simulink model "DoublePendulumPM"  (R2023b)
settings: Solver=FixedStepAuto  StartTime=0.0  StopTime=5  FixedStep=0.0001  RelTol=1e-3
values from neighbouring files (symbols this model uses):
  an1 = pm.Constants.r_0 / pm.Constants.l_1    [Constants.m]    (also in DoublePendulumPM_ParamSet.m = 1.5)
  an2 = pm.Constants.r_0 / pm.Constants.l_2    [Constants.m]    (also in DoublePendulumPM_ParamSet.m = 3)
  cn1 = pm.Constants.c_1 / (pm.Constants.m_1 * pm.Constants.l_1^2)    [Constants.m]    (also in DoublePendulumPM_ParamSet.m = 0.025)
  cn2 = pm.Constants.c_2 / (pm.Constants.m_2 * pm.Constants.l_2^2)    [Constants.m]    (also in DoublePendulumPM_ParamSet.m = 0.1)
  dt = 0.01    [Constants.m]    (also in DoublePendulumPM_ParamSet.m)
  l_1 = 0.2    [Constants.m]    (also in DoublePendulumPM_ParamSet.m)
  l_2 = 0.1    [Constants.m]    (also in DoublePendulumPM_ParamSet.m)
  m_1 = 1    [Constants.m]    (also in DoublePendulumPM_ParamSet.m)
  m_2 = 1    [Constants.m]    (also in DoublePendulumPM_ParamSet.m)
  N = 181    [Constants.m]
  r_0 = 0.3    [Constants.m]    (also in DoublePendulumPM_ParamSet.m)
  s = [10000.0; 10000.0; 80000.0; 5000.0; 80000.0; 5000.0]    [Constants.m]
  wn1 = pm.Constants.g   / pm.Constants.l_1    [Constants.m]    (also in DoublePendulumPM_ParamSet.m = 49.03325)
  wn2 = pm.Constants.g   / pm.Constants.l_2    [Constants.m]    (also in DoublePendulumPM_ParamSet.m = 98.0665)
undefined symbols (not defined in the file or in its folder): L, X, Y, Z
libraries: sm_lib x28, nesl_utility x9
settings Model: Creator=s0612  LastModifiedBy=0484476

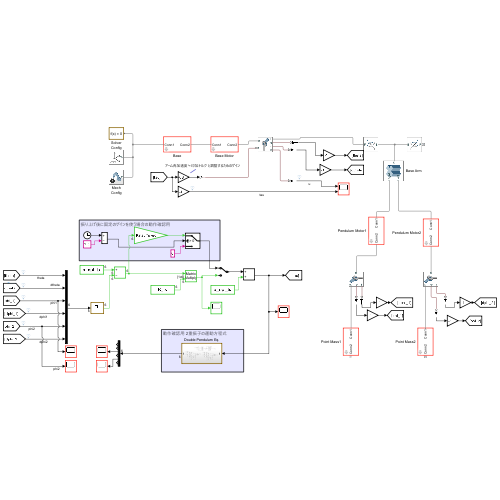
[thumbnail: Simulink's stored preview of the top-level diagram]
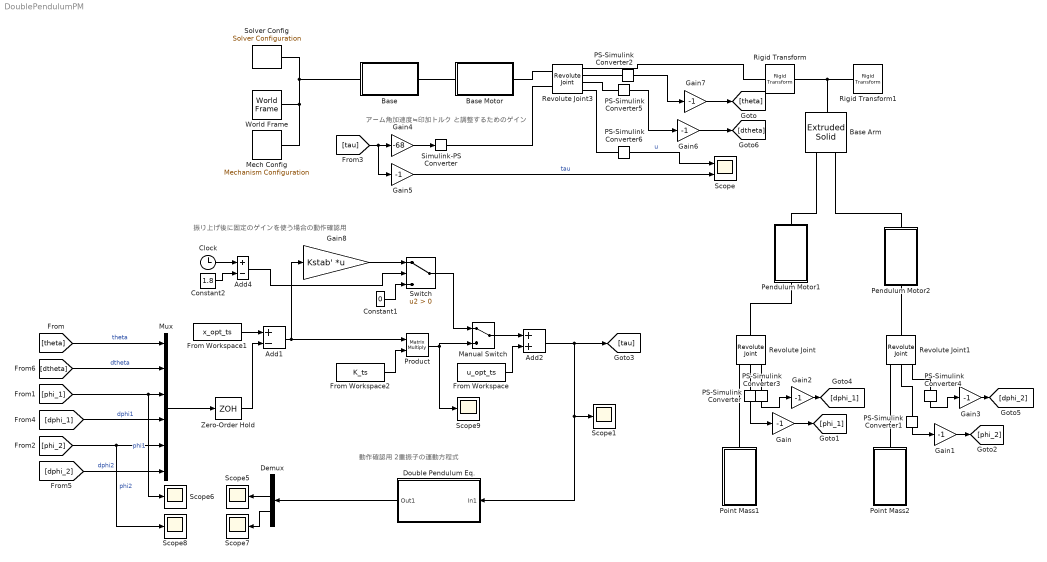
== system DoublePendulumPM ==
  note: アーム角加速度≒印加トルク と調整するためのゲイン
  note: 動作確認用 2重振子の運動方程式
  note: 振り上げ後に固定のゲインを使う場合の動作確認用
  Add1 : Sum  Inputs=+-
  Add2 : Sum
  Add4 : Sum  Inputs=+-
  Base : Subsystem  mask{L=0.2, R=0.2, rho=1000, rgb=[0.5 0.5 0.5]}
      mask prompts: L "Length[m]"; R "Radius[m]"; rho "Density[kg/m^3]"; rgb "Color (R G B)"
      mask DialogControl ParameterGroupVar Prompt: パラメーター
  Base Arm : sm_lib/Body Elements/Extruded Solid  GraphicAmbientColor=[0.15 0.15 0.15 1.0]  BasedOnType=Density  CenterOfMass=[0 0 0]  CenterOfMassUnits=m  GraphicDiffuseColor=[0.5 0.5 0.5]  ExportConvexHullGeometry=off  ExtrusionCrossSection=[r_0 0.04; 0 0.06; -r_0 0.04; -r_0 -0.04; 0 -0.06; r_0 -0.04]  ExtrusionCrossSectionUnits=m  Density=1000*1000  DensityUnits=kg/m^3  DoExposeReferenceFrame=on  GraphicEmissiveColor=[0.0 0.0 0.0 1.0]  ExportEntireGeometry=off  ExtrusionLength=0.04  ExtrusionLengthUnits=m  ExtrusionType=General  SerializedFrames=<Frames><Frame><Id>Frame1</Id><Value><Name>Right</Name><Origin><Source>GeometricFeature</Source><FeatureName>side surface 6</FeatureName></Origin><PrimaryAxis><DefinedDirection>+Z</DefinedDirection><Source>ReferenceFrame</Source><SourceDirection>+X</SourceDirection><FeatureName></FeatureName></PrimaryAxis><SecondaryAxis><DefinedDirection>+Y</DefinedDirection><Source>ReferenceFrame</Source><SourceDirection>+Y</SourceDirection><FeatureName></FeatureName></SecondaryAxis></Value></Frame><Frame><Id>Frame2</Id><Value><Name>Left</Name><Origin><Source>GeometricFeature</Source><FeatureName>side surface 3</FeatureName></Origin><PrimaryAxis><DefinedDirection>+Z</DefinedDirection><Source>ReferenceFrame</Source><SourceDirection>-X</SourceDirection><FeatureName></FeatureName></PrimaryAxis><SecondaryAxis><DefinedDirection>+Y</DefinedDirection><Source>ReferenceFrame</Source><SourceDirection>-Y</SourceDirection><FeatureName></FeatureName></SecondaryAxis></Value></Frame></Frames>  MarkerShape=Sphere  MarkerSize=10  GraphicType=FromGeometry  InertiaType=CalculateFromGeometry  Mass=1  MassUnits=kg  MomentsOfInertia=[1 1 1]  MomentsOfInertiaUnits=kg*m^2  PolygonNumSides=6  GraphicOpacity=1.0  PolygonOuterRadius=1  PolygonOuterRadiusUnits=m  ProductsOfInertia=[0 0 0]  ProductsOfInertiaUnits=kg*m^2  GraphicShininess=75  GraphicSpecularColor=[0.5 0.5 0.5 1.0]  GraphicVisPropType=SimpleVisualProperties
  Base Motor : Subsystem  mask{L=0.02, R=0.1, rho=1000, rgb=[0.5 0.5 0]}
      mask prompts: L "Length[m]"; R "Radius[m]"; rho "Density[kg/m^3]"; rgb "Color (R G B)"
      mask DialogControl ParameterGroupVar Prompt: パラメーター
  Clock : Clock
  Constant1 : Constant  Value=0
  Constant2 : Constant  Value=1.8
  Demux : Demux  Outputs=6
  Double Pendulum Eq. : Subsystem
  From Workspace : FromWorkspace  VariableName=u_opt_ts  SampleTime=0.01
  From Workspace1 : FromWorkspace  VariableName=x_opt_ts  SampleTime=dt  OutputAfterFinalValue=Holding final value
  From Workspace2 : FromWorkspace  VariableName=K_ts  SampleTime=dt  OutputAfterFinalValue=Holding final value
  Gain{,1..3,5..7} (7 alike) : Gain  Gain=-1
  Gain4 : Gain  Gain=-68
  Gain8 : Gain  Gain=Kstab'  Multiplication=Matrix(K*u) (u vector)
  Manual Switch : ManualSwitch
  Mech Config : sm_lib/Utilities/Mechanism Configuration  UniformGravity=Constant  GravityVector=[0 0 -9.80665]  GravityVectorUnits=m/s^2  LinearizationDelta=0.001  JointModeTransitionNonlinearIterations=2
  Mux : Mux  Inputs=6
  PS-Simulink Converter{,1..6} (7 alike) : nesl_utility/PS-Simulink Converter  PhysicalDomain=network_engine_domain  SubClassName=ps_output  LeftPortType=input  RightPortType=output  PseudoPeriodic=off  Frequencies=[]  VectorFormat=inherit  Unit=inherit  AffineConversion=off
  Pendulum Motor1 : Subsystem  mask{L=0.005, R=0.02, rho=0, rgb=[0.5 0.5 0]}
      mask prompts: L "Length[m]"; R "Radius[m]"; rho "Density[kg/m^3]"; rgb "Color (R G B)"
      mask DialogControl ParameterGroupVar Prompt: パラメーター
  Pendulum Motor2 : Subsystem  mask{L=0.005, R=0.02, rho=0, rgb=[0.5 0.5 0]}
      mask prompts: L "Length[m]"; R "Radius[m]"; rho "Density[kg/m^3]"; rgb "Color (R G B)"
      mask DialogControl ParameterGroupVar Prompt: パラメーター
  Point Mass1 : Subsystem  mask{L=l_1, M=m_1, rgb=[1 0.5 0]}
      mask prompts: L "Length[m]"; M "Weight[kg]"; rgb "Color (R G B)"
      mask DialogControl ParameterGroupVar Prompt: パラメーター
  Point Mass2 : Subsystem  mask{L=l_2, M=m_2, rgb=[0 1 0.5]}
      mask prompts: L "Length[m]"; M "Weight[kg]"; rgb "Color (R G B)"
      mask DialogControl ParameterGroupVar Prompt: パラメーター
  Product : Product  Multiplication=Matrix(*)
  Revolute Joint : sm_lib/Joints/Revolute Joint  JointMode=Normal  SenseConstraintForce=off  SenseConstraintForceX=off  SenseConstraintForceY=off  SenseConstraintForceZ=off  SenseConstraintTorque=off  SenseConstraintTorqueX=off  SenseConstraintTorqueY=off  SenseConstraintTorqueZ=off  SenseTotalForce=off  SenseTotalForceX=off  SenseTotalForceY=off  SenseTotalForceZ=off  SenseTotalTorque=off  SenseTotalTorqueX=off  SenseTotalTorqueY=off  SenseTotalTorqueZ=off  CompositeWrenchDir=FollowerOnBase  CompositeWrenchFrame=BaseFrame  EquilibriumPosition=0  EquilibriumPositionUnits=deg  SpringStiffness=0  SpringStiffnessUnits=N*m/deg  DampingCoefficient=c_1  DampingCoefficientUnits=N*m*s/rad  TorqueActuationMode=NoTorque  MotionActuationMode=ComputedMotion  SensePosition=on  SenseVelocity=on  SenseAcceleration=off  SenseTorqueForce=off  SenseLowerLimitTorqueForce=off  SenseUpperLimitTorqueForce=off  LowerLimitSpecify=off  LowerLimitBound=-90  LowerLimitBoundUnits=deg  LowerLimitStiffness=1e4  LowerLimitStiffnessUnits=N*m/deg  LowerLimitDamping=10  LowerLimitDampingUnits=N*m/(deg/s)  LowerLimitTransitionRegionWidth=0.1  LowerLimitTransitionRegionWidthUnits=deg  UpperLimitSpecify=off  UpperLimitBound=90  UpperLimitBoundUnits=deg  UpperLimitStiffness=1e4  UpperLimitStiffnessUnits=N*m/deg  UpperLimitDamping=10  UpperLimitDampingUnits=N*m/(deg/s)  UpperLimitTransitionRegionWidth=0.1  UpperLimitTransitionRegionWidthUnits=deg  PositionTargetSpecify=off  PositionTargetPriority=High  PositionTargetValue=90  PositionTargetValueUnits=deg  VelocityTargetSpecify=off  VelocityTargetPriority=High  VelocityTargetValue=0  VelocityTargetValueUnits=deg/s
  Revolute Joint1 : sm_lib/Joints/Revolute Joint  JointMode=Normal  SenseConstraintForce=off  SenseConstraintForceX=off  SenseConstraintForceY=off  SenseConstraintForceZ=off  SenseConstraintTorque=off  SenseConstraintTorqueX=off  SenseConstraintTorqueY=off  SenseConstraintTorqueZ=off  SenseTotalForce=off  SenseTotalForceX=off  SenseTotalForceY=off  SenseTotalForceZ=off  SenseTotalTorque=off  SenseTotalTorqueX=off  SenseTotalTorqueY=off  SenseTotalTorqueZ=off  CompositeWrenchDir=FollowerOnBase  CompositeWrenchFrame=BaseFrame  EquilibriumPosition=0  EquilibriumPositionUnits=deg  SpringStiffness=0  SpringStiffnessUnits=N*m/deg  DampingCoefficient=c_2  DampingCoefficientUnits=N*m*s/rad  TorqueActuationMode=NoTorque  MotionActuationMode=ComputedMotion  SensePosition=on  SenseVelocity=on  SenseAcceleration=off  SenseTorqueForce=off  SenseLowerLimitTorqueForce=off  SenseUpperLimitTorqueForce=off  LowerLimitSpecify=off  LowerLimitBound=-90  LowerLimitBoundUnits=deg  LowerLimitStiffness=1e4  LowerLimitStiffnessUnits=N*m/deg  LowerLimitDamping=10  LowerLimitDampingUnits=N*m/(deg/s)  LowerLimitTransitionRegionWidth=0.1  LowerLimitTransitionRegionWidthUnits=deg  UpperLimitSpecify=off  UpperLimitBound=90  UpperLimitBoundUnits=deg  UpperLimitStiffness=1e4  UpperLimitStiffnessUnits=N*m/deg  UpperLimitDamping=10  UpperLimitDampingUnits=N*m/(deg/s)  UpperLimitTransitionRegionWidth=0.1  UpperLimitTransitionRegionWidthUnits=deg  PositionTargetSpecify=off  PositionTargetPriority=High  PositionTargetValue=90  PositionTargetValueUnits=deg  VelocityTargetSpecify=off  VelocityTargetPriority=High  VelocityTargetValue=0  VelocityTargetValueUnits=deg/s
  Revolute Joint3 : sm_lib/Joints/Revolute Joint  JointMode=Normal  SenseConstraintForce=off  SenseConstraintForceX=off  SenseConstraintForceY=off  SenseConstraintForceZ=off  SenseConstraintTorque=off  SenseConstraintTorqueX=off  SenseConstraintTorqueY=off  SenseConstraintTorqueZ=off  SenseTotalForce=off  SenseTotalForceX=off  SenseTotalForceY=off  SenseTotalForceZ=off  SenseTotalTorque=off  SenseTotalTorqueX=off  SenseTotalTorqueY=off  SenseTotalTorqueZ=off  CompositeWrenchDir=BaseOnFollower  CompositeWrenchFrame=FollowerFrame  EquilibriumPosition=0  EquilibriumPositionUnits=deg  SpringStiffness=0  SpringStiffnessUnits=N*m/deg  DampingCoefficient=0  DampingCoefficientUnits=N*m/(deg/s)  TorqueActuationMode=InputTorque  MotionActuationMode=ComputedMotion  SensePosition=on  SenseVelocity=on  SenseAcceleration=on  SenseTorqueForce=off  SenseLowerLimitTorqueForce=off  SenseUpperLimitTorqueForce=off  LowerLimitSpecify=off  LowerLimitBound=-90  LowerLimitBoundUnits=deg  LowerLimitStiffness=1e4  LowerLimitStiffnessUnits=N*m/deg  LowerLimitDamping=10  LowerLimitDampingUnits=N*m/(deg/s)  LowerLimitTransitionRegionWidth=0.1  LowerLimitTransitionRegionWidthUnits=deg  UpperLimitSpecify=off  UpperLimitBound=90  UpperLimitBoundUnits=deg  UpperLimitStiffness=1e4  UpperLimitStiffnessUnits=N*m/deg  UpperLimitDamping=10  UpperLimitDampingUnits=N*m/(deg/s)  UpperLimitTransitionRegionWidth=0.1  UpperLimitTransitionRegionWidthUnits=deg  PositionTargetSpecify=off  PositionTargetPriority=High  PositionTargetValue=0  PositionTargetValueUnits=deg  VelocityTargetSpecify=off  VelocityTargetPriority=High  VelocityTargetValue=0  VelocityTargetValueUnits=deg/s
  Rigid Transform : sm_lib/Frames and Transforms/Rigid Transform  TranslationMethod=StandardAxis  TranslationStandardOffset=0.04/2  TranslationStandardOffsetUnits=m  TranslationStandardAxis=-Z  TranslationCartesianOffset=[0 0 0]  TranslationCartesianOffsetUnits=m  TranslationROffset=0  TranslationROffsetUnits=m  TranslationZOffset=0  TranslationZOffsetUnits=m  TranslationThetaOffset=0  TranslationThetaOffsetUnits=deg  RotationMethod=None  RotationAngleUnits=deg  RotationStandardAxis=-X  RotationAngle=L/2  RotationArbitraryAxis=[0 0 1]  FollAlignAxisA=-X  BaseAlignAxisA=+Y  FollAlignAxisB=+Y  BaseAlignAxisB=+Z  RotationSequenceAxes=FollowerAxes  RotationSequence=XYX  RotationSequenceAngles=[0 0 0]  RotationSequenceAnglesUnits=deg  RotationMatrix=[1 0 0; 0 1 0; 0 0 1]  Quaternion=[1 0 0 0]
  Rigid Transform1 : sm_lib/Frames and Transforms/Rigid Transform  TranslationMethod=StandardAxis  TranslationStandardOffset=0.04/2  TranslationStandardOffsetUnits=m  TranslationStandardAxis=+Z  TranslationCartesianOffset=[0 0 0]  TranslationCartesianOffsetUnits=m  TranslationROffset=0  TranslationROffsetUnits=m  TranslationZOffset=0  TranslationZOffsetUnits=m  TranslationThetaOffset=0  TranslationThetaOffsetUnits=deg  RotationMethod=None  RotationAngleUnits=deg  RotationStandardAxis=-X  RotationAngle=L/2  RotationArbitraryAxis=[0 0 1]  FollAlignAxisA=-X  BaseAlignAxisA=+Y  FollAlignAxisB=+Y  BaseAlignAxisB=+Z  RotationSequenceAxes=FollowerAxes  RotationSequence=XYX  RotationSequenceAngles=[0 0 0]  RotationSequenceAnglesUnits=deg  RotationMatrix=[1 0 0; 0 1 0; 0 0 1]  Quaternion=[1 0 0 0]
  Scope : Scope  NumInputPorts=2
  Scope{1,5..9} (6 alike) : Scope
  Simulink-PS Converter : nesl_utility/Simulink-PS Converter  PhysicalDomain=network_engine_domain  SubClassName=ps_input  LeftPortType=input  RightPortType=output  PseudoPeriodic=off  Frequencies=[]  NoiseDistribution=none  NoiseParameters=[]  Unit=1  AffineConversion=off  FilteringAndDerivatives=provide  SimscapeFilterOrder=1  InputFilterTimeConstant=0.001  UdotUserProvided=0
  Solver Config : nesl_utility/Solver Configuration  PhysicalDomain=network_engine_domain  SubClassName=solver  LeftPortType=input  RightPortType=generic  Tones=[]  Harmonics=[]  SimulateNoise=off  Profile=off  UseLocalSampling=off  EnableSwitchedLinearOptims=on  FrequencyDomain=off  UseCCode=off  RelTol=0.001  AbsTol=1e-06  MinStep=1e-09  ToWorkspace=off  RevertToSquareIcSolve=off  NumHomotopyIterations=100  PhasorMode=off  PhasorModeNumHarmonics=1  ConsistencySolver=NEWTON_FTOL  IndexReductionMethod=DerivativeReplacement  DoDC=off  ResidualTolerance=1e-09  ConsistencyTolSource=GLOBAL  ConsistencyAbsTol=0.001  ConsistencyRelTol=0.001  ConsistencyTolFactor=0.001  UseLocalSolver=off  LocalSolverChoice=NE_BACKWARD_EULER_ADVANCER  ResolveIndetEquations=on  FunctionEvalNumThread=1  LocalSolverSampleTime=0.001  DoFixedCost=off  MaxNonlinIter=3  MaxModeIter=2  ComputeImpulses=off  ImpulseIterations=2  LinearAlgebra=Sparse  LinearAlgebraNumThread=0  EquationFormulation=NE_TIME_EF  DelaysMemoryBudget=1024  AutomaticFiltering=on  FilteringTimeConstant=0.001  PartitionStorageMethod=AS_NEEDED  PartitionMemoryBudget=1024  PartitionMethod=FAST  MultibodyUseLocalSolver=off  MultibodyLocalSolverChoice=ODE1  MultibodyLocalSolverSampleTime=0.001
  Switch : Switch  Criteria=u2 > Threshold  SaturateOnIntegerOverflow=off  InputSameDT=off
  World Frame : sm_lib/Frames and Transforms/World Frame
  Zero-Order Hold : ZeroOrderHold  SampleTime=dt
  wires:
  PS-Simulink Converter2/1 -> Gain7/1
  PS-Simulink Converter/1 -> Gain/1
  Add2/1 -> Scope1/1, Double Pendulum Eq./1(In1), [tau]
  Gain/1 -> [phi_1]
  Gain2/1 -> [dphi_1]
  PS-Simulink Converter3/1 -> Gain2/1
  Gain1/1 -> [phi_2]
  PS-Simulink Converter1/1 -> Gain1/1
  Gain3/1 -> [dphi_2]
  PS-Simulink Converter4/1 -> Gain3/1
  [phi_1] -> Scope6/1, Mux/3  "phi1"
  [dphi_1] -> Mux/4  "dphi1"
  [phi_2] -> Scope8/1, Mux/5  "phi2"
  [dphi_2] -> Mux/6  "dphi2"
  Add1/1 -> Product/1, Gain8/1
  PS-Simulink Converter5/1 -> Gain6/1
  [dtheta] -> Mux/2  "dtheta"
  [theta] -> Mux/1  "theta"
  PS-Simulink Converter6/1 -> Scope/1  "u"
  [tau] -> Gain5/1, Gain4/1
  Demux/3 -> Scope5/1
  Gain4/1 -> Simulink-PS Converter/1
  Demux/5 -> Scope7/1
  Add4/1 -> Switch/2
  Constant1/1 -> Switch/3
  Clock/1 -> Add4/1
  Constant2/1 -> Add4/2
  Gain6/1 -> [dtheta]
  Gain7/1 -> [theta]
  Gain8/1 -> Switch/1
  Product/1 -> Manual Switch/2, Scope9/1
  Gain5/1 -> Scope/2  "tau"
  Double Pendulum Eq./1(Out1) -> Demux/1
  Zero-Order Hold/1 -> Add1/2
  From Workspace/1 -> Add2/2
  From Workspace1/1 -> Add1/1
  Mux/1 -> Zero-Order Hold/1
  From Workspace2/1 -> Product/2
  Manual Switch/1 -> Add2/1
  Switch/1 -> Manual Switch/1
  connections:
  World Frame/RConn1 -- Base/LConn1 -- Solver Config/RConn1 -- Mech Config/RConn1
  Base Motor/LConn1 -- Base/RConn1
  Rigid Transform1/LConn1 -- Rigid Transform/LConn1 -- Base Arm/RConn1
  Revolute Joint3/LConn1 -- Base Motor/RConn1
  Point Mass2/LConn1 -- Revolute Joint1/RConn1
  Pendulum Motor1/LConn1 -- Base Arm/LConn1
  Pendulum Motor2/LConn1 -- Base Arm/LConn2
  Revolute Joint/LConn1 -- Pendulum Motor1/RConn1
  Revolute Joint/RConn1 -- Point Mass1/LConn1
  Revolute Joint1/LConn1 -- Pendulum Motor2/RConn1
  Rigid Transform/RConn1 -- Revolute Joint3/RConn1
  Simulink-PS Converter/RConn1 -- Revolute Joint3/LConn2
  PS-Simulink Converter/LConn1 -- Revolute Joint/RConn2
  Revolute Joint1/RConn2 -- PS-Simulink Converter1/LConn1
  PS-Simulink Converter2/LConn1 -- Revolute Joint3/RConn2
  PS-Simulink Converter3/LConn1 -- Revolute Joint/RConn3
  PS-Simulink Converter4/LConn1 -- Revolute Joint1/RConn3
  PS-Simulink Converter5/LConn1 -- Revolute Joint3/RConn3
  PS-Simulink Converter6/LConn1 -- Revolute Joint3/RConn4

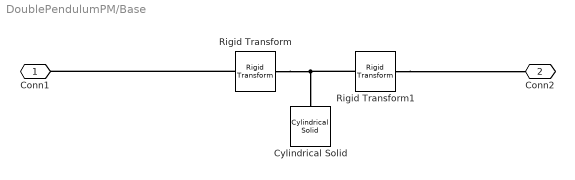
== system DoublePendulumPM/Base ==
  Cylindrical Solid : sm_lib/Body Elements/Cylindrical Solid  GraphicAmbientColor=[0.15 0.15 0.15 1.0]  BasedOnType=Density  CenterOfMass=[0 0 0]  CenterOfMassUnits=m  GraphicDiffuseColor=rgb  CylinderLength=L  CylinderLengthUnits=m  CylinderRadius=R  CylinderRadiusUnits=m  Density=rho  DensityUnits=kg/m^3  DoExposeReferenceFrame=on  GraphicEmissiveColor=[0.0 0.0 0.0 1.0]  ExportEntireGeometry=off  SerializedFrames=<Frames/>  MarkerShape=Sphere  MarkerSize=10  GraphicType=FromGeometry  InertiaType=CalculateFromGeometry  Mass=1  MassUnits=kg  MomentsOfInertia=[1 1 1]  MomentsOfInertiaUnits=kg*m^2  GraphicOpacity=1.0  ProductsOfInertia=[0 0 0]  ProductsOfInertiaUnits=kg*m^2  GraphicShininess=75  GraphicSpecularColor=[0.5 0.5 0.5 1.0]  GraphicVisPropType=SimpleVisualProperties
  Rigid Transform : sm_lib/Frames and Transforms/Rigid Transform  TranslationMethod=StandardAxis  TranslationStandardOffset=L/2  TranslationStandardOffsetUnits=m  TranslationStandardAxis=-Z  TranslationCartesianOffset=[0 0 0]  TranslationCartesianOffsetUnits=m  TranslationROffset=0  TranslationROffsetUnits=m  TranslationZOffset=0  TranslationZOffsetUnits=m  TranslationThetaOffset=0  TranslationThetaOffsetUnits=deg  RotationMethod=None  RotationAngleUnits=deg  RotationStandardAxis=-X  RotationAngle=L/2  RotationArbitraryAxis=[0 0 1]  FollAlignAxisA=-X  BaseAlignAxisA=+Y  FollAlignAxisB=+Y  BaseAlignAxisB=+Z  RotationSequenceAxes=FollowerAxes  RotationSequence=XYX  RotationSequenceAngles=[0 0 0]  RotationSequenceAnglesUnits=deg  RotationMatrix=[1 0 0; 0 1 0; 0 0 1]  Quaternion=[1 0 0 0]
  Rigid Transform1 : sm_lib/Frames and Transforms/Rigid Transform  TranslationMethod=StandardAxis  TranslationStandardOffset=L/2  TranslationStandardOffsetUnits=m  TranslationStandardAxis=+Z  TranslationCartesianOffset=[0 0 0]  TranslationCartesianOffsetUnits=m  TranslationROffset=0  TranslationROffsetUnits=m  TranslationZOffset=0  TranslationZOffsetUnits=m  TranslationThetaOffset=0  TranslationThetaOffsetUnits=deg  RotationMethod=None  RotationAngleUnits=deg  RotationStandardAxis=-X  RotationAngle=L/2  RotationArbitraryAxis=[0 0 1]  FollAlignAxisA=-X  BaseAlignAxisA=+Y  FollAlignAxisB=+Y  BaseAlignAxisB=+Z  RotationSequenceAxes=FollowerAxes  RotationSequence=XYX  RotationSequenceAngles=[0 0 0]  RotationSequenceAnglesUnits=deg  RotationMatrix=[1 0 0; 0 1 0; 0 0 1]  Quaternion=[1 0 0 0]
  Conn1 : PMIOPort  Side=Left
  Conn2 : PMIOPort  Port=2  Side=Right
  connections:
  Rigid Transform/LConn1 -- Rigid Transform1/LConn1 -- Cylindrical Solid/RConn1
  Rigid Transform1/RConn1 -- Conn2/RConn1
  Rigid Transform/RConn1 -- Conn1/RConn1

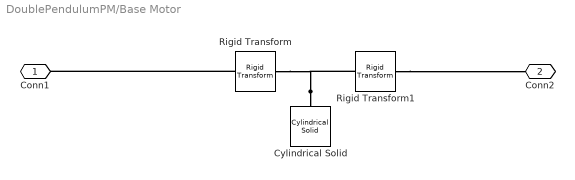
== system DoublePendulumPM/Base Motor ==
  Cylindrical Solid : sm_lib/Body Elements/Cylindrical Solid  GraphicAmbientColor=[0.15 0.15 0.15 1.0]  BasedOnType=Density  CenterOfMass=[0 0 0]  CenterOfMassUnits=m  GraphicDiffuseColor=rgb  CylinderLength=L  CylinderLengthUnits=m  CylinderRadius=R  CylinderRadiusUnits=m  Density=rho  DensityUnits=kg/m^3  DoExposeReferenceFrame=on  GraphicEmissiveColor=[0.0 0.0 0.0 1.0]  ExportEntireGeometry=off  SerializedFrames=<Frames/>  MarkerShape=Sphere  MarkerSize=10  GraphicType=FromGeometry  InertiaType=CalculateFromGeometry  Mass=1  MassUnits=kg  MomentsOfInertia=[1 1 1]  MomentsOfInertiaUnits=kg*m^2  GraphicOpacity=1.0  ProductsOfInertia=[0 0 0]  ProductsOfInertiaUnits=kg*m^2  GraphicShininess=75  GraphicSpecularColor=[0.5 0.5 0.5 1.0]  GraphicVisPropType=SimpleVisualProperties
  Rigid Transform : sm_lib/Frames and Transforms/Rigid Transform  TranslationMethod=StandardAxis  TranslationStandardOffset=L/2  TranslationStandardOffsetUnits=m  TranslationStandardAxis=-Z  TranslationCartesianOffset=[0 0 0]  TranslationCartesianOffsetUnits=m  TranslationROffset=0  TranslationROffsetUnits=m  TranslationZOffset=0  TranslationZOffsetUnits=m  TranslationThetaOffset=0  TranslationThetaOffsetUnits=deg  RotationMethod=None  RotationAngleUnits=deg  RotationStandardAxis=-X  RotationAngle=L/2  RotationArbitraryAxis=[0 0 1]  FollAlignAxisA=-X  BaseAlignAxisA=+Y  FollAlignAxisB=+Y  BaseAlignAxisB=+Z  RotationSequenceAxes=FollowerAxes  RotationSequence=XYX  RotationSequenceAngles=[0 0 0]  RotationSequenceAnglesUnits=deg  RotationMatrix=[1 0 0; 0 1 0; 0 0 1]  Quaternion=[1 0 0 0]
  Rigid Transform1 : sm_lib/Frames and Transforms/Rigid Transform  TranslationMethod=StandardAxis  TranslationStandardOffset=L/2  TranslationStandardOffsetUnits=m  TranslationStandardAxis=+Z  TranslationCartesianOffset=[0 0 0]  TranslationCartesianOffsetUnits=m  TranslationROffset=0  TranslationROffsetUnits=m  TranslationZOffset=0  TranslationZOffsetUnits=m  TranslationThetaOffset=0  TranslationThetaOffsetUnits=deg  RotationMethod=None  RotationAngleUnits=deg  RotationStandardAxis=-X  RotationAngle=L/2  RotationArbitraryAxis=[0 0 1]  FollAlignAxisA=-X  BaseAlignAxisA=+Y  FollAlignAxisB=+Y  BaseAlignAxisB=+Z  RotationSequenceAxes=FollowerAxes  RotationSequence=XYX  RotationSequenceAngles=[0 0 0]  RotationSequenceAnglesUnits=deg  RotationMatrix=[1 0 0; 0 1 0; 0 0 1]  Quaternion=[1 0 0 0]
  Conn1 : PMIOPort  Side=Left
  Conn2 : PMIOPort  Port=2  Side=Right
  connections:
  Cylindrical Solid/RConn1 -- Rigid Transform/LConn1 -- Rigid Transform1/LConn1
  Rigid Transform1/RConn1 -- Conn2/RConn1
  Rigid Transform/RConn1 -- Conn1/RConn1

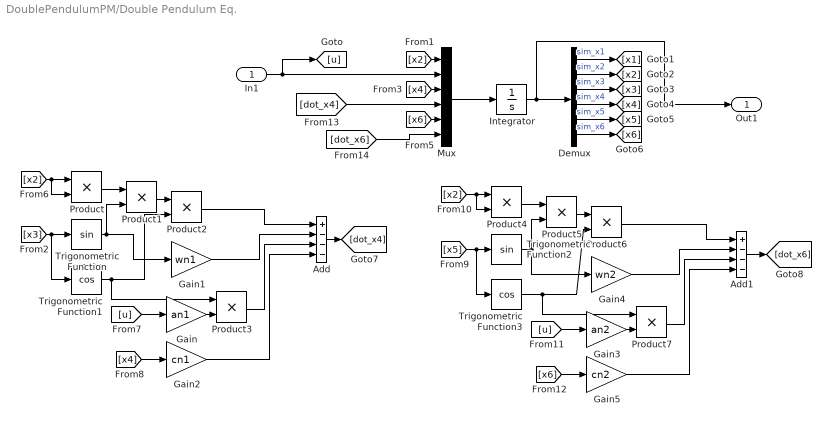
== system DoublePendulumPM/Double Pendulum Eq. ==
  In1 : Inport
  Add : Sum  Inputs=+---
  Add1 : Sum  Inputs=+---
  Demux : Demux  Outputs=6
  Gain : Gain  Gain=an1
  Gain1 : Gain  Gain=wn1
  Gain2 : Gain  Gain=cn1
  Gain3 : Gain  Gain=an2
  Gain4 : Gain  Gain=wn2
  Gain5 : Gain  Gain=cn2
  Integrator : Integrator  InitialCondition=[0 0 0 0 0 0]
  Mux : Mux  Inputs=6
  Product{,1..7} (8 alike) : Product
  Trigonometric Function : Trigonometry
  Trigonometric Function1 : Trigonometry  Operator=cos
  Trigonometric Function2 : Trigonometry
  Trigonometric Function3 : Trigonometry  Operator=cos
  Out1 : Outport
  wires:
  In1/1 -> Mux/2, [u]
  Integrator/1 -> Out1/1, Demux/1
  Mux/1 -> Integrator/1
  Product/1 -> Product1/1
  Product1/1 -> Product2/1
  Product2/1 -> Add/1
  Trigonometric Function/1 -> Product1/2, Gain1/1
  Trigonometric Function1/1 -> Product3/1, Product2/2
  Demux/1 -> [x1]  "sim_x1"
  Demux/2 -> [x2]  "sim_x2"
  Demux/3 -> [x3]  "sim_x3"
  Demux/4 -> [x4]  "sim_x4"
  Demux/5 -> [x5]  "sim_x5"
  Demux/6 -> [x6]  "sim_x6"
  [x2] -> Mux/1
  [x6] -> Mux/5
  [x4] -> Mux/3
  [x3] -> Trigonometric Function1/1, Trigonometric Function/1
  [x2] -> Product/2, Product/1
  [u] -> Gain/1
  Gain/1 -> Product3/2
  Gain1/1 -> Add/2
  Product3/1 -> Add/3
  Gain2/1 -> Add/4
  [x4] -> Gain2/1
  Gain3/1 -> Product7/2
  [x5] -> Trigonometric Function3/1, Trigonometric Function2/1
  Product7/1 -> Add1/3
  Product5/1 -> Product6/1
  Product4/1 -> Product5/1
  Product6/1 -> Add1/1
  Gain5/1 -> Add1/4
  [x2] -> Product4/2, Product4/1
  Trigonometric Function2/1 -> Product5/2, Gain4/1
  [x6] -> Gain5/1
  Gain4/1 -> Add1/2
  [u] -> Gain3/1
  Trigonometric Function3/1 -> Product7/1, Product6/2
  Add/1 -> [dot_x4]
  [dot_x4] -> Mux/4
  Add1/1 -> [dot_x6]
  [dot_x6] -> Mux/6

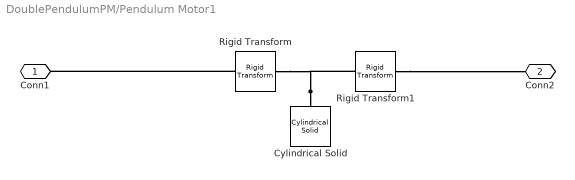
== system DoublePendulumPM/Pendulum Motor1 ==
  Cylindrical Solid : sm_lib/Body Elements/Cylindrical Solid  GraphicAmbientColor=[0.15 0.15 0.15 1.0]  BasedOnType=Density  CenterOfMass=[0 0 0]  CenterOfMassUnits=m  GraphicDiffuseColor=rgb  CylinderLength=L  CylinderLengthUnits=m  CylinderRadius=R  CylinderRadiusUnits=m  Density=rho  DensityUnits=kg/m^3  DoExposeReferenceFrame=on  GraphicEmissiveColor=[0.0 0.0 0.0 1.0]  ExportEntireGeometry=off  SerializedFrames=<Frames/>  MarkerShape=Sphere  MarkerSize=10  GraphicType=FromGeometry  InertiaType=CalculateFromGeometry  Mass=1  MassUnits=kg  MomentsOfInertia=[1 1 1]  MomentsOfInertiaUnits=kg*m^2  GraphicOpacity=1.0  ProductsOfInertia=[0 0 0]  ProductsOfInertiaUnits=kg*m^2  GraphicShininess=75  GraphicSpecularColor=[0.5 0.5 0.5 1.0]  GraphicVisPropType=SimpleVisualProperties
  Rigid Transform : sm_lib/Frames and Transforms/Rigid Transform  TranslationMethod=StandardAxis  TranslationStandardOffset=L/2  TranslationStandardOffsetUnits=m  TranslationStandardAxis=-Z  TranslationCartesianOffset=[0 0 0]  TranslationCartesianOffsetUnits=m  TranslationROffset=0  TranslationROffsetUnits=m  TranslationZOffset=0  TranslationZOffsetUnits=m  TranslationThetaOffset=0  TranslationThetaOffsetUnits=deg  RotationMethod=None  RotationAngleUnits=deg  RotationStandardAxis=-X  RotationAngle=L/2  RotationArbitraryAxis=[0 0 1]  FollAlignAxisA=-X  BaseAlignAxisA=+Y  FollAlignAxisB=+Y  BaseAlignAxisB=+Z  RotationSequenceAxes=FollowerAxes  RotationSequence=XYX  RotationSequenceAngles=[0 0 0]  RotationSequenceAnglesUnits=deg  RotationMatrix=[1 0 0; 0 1 0; 0 0 1]  Quaternion=[1 0 0 0]
  Rigid Transform1 : sm_lib/Frames and Transforms/Rigid Transform  TranslationMethod=StandardAxis  TranslationStandardOffset=L/2  TranslationStandardOffsetUnits=m  TranslationStandardAxis=+Z  TranslationCartesianOffset=[0 0 0]  TranslationCartesianOffsetUnits=m  TranslationROffset=0  TranslationROffsetUnits=m  TranslationZOffset=0  TranslationZOffsetUnits=m  TranslationThetaOffset=0  TranslationThetaOffsetUnits=deg  RotationMethod=None  RotationAngleUnits=deg  RotationStandardAxis=-X  RotationAngle=L/2  RotationArbitraryAxis=[0 0 1]  FollAlignAxisA=-X  BaseAlignAxisA=+Y  FollAlignAxisB=+Y  BaseAlignAxisB=+Z  RotationSequenceAxes=FollowerAxes  RotationSequence=XYX  RotationSequenceAngles=[0 0 0]  RotationSequenceAnglesUnits=deg  RotationMatrix=[1 0 0; 0 1 0; 0 0 1]  Quaternion=[1 0 0 0]
  Conn1 : PMIOPort  Side=Left
  Conn2 : PMIOPort  Port=2  Side=Right
  connections:
  Cylindrical Solid/RConn1 -- Rigid Transform/LConn1 -- Rigid Transform1/LConn1
  Rigid Transform1/RConn1 -- Conn2/RConn1
  Rigid Transform/RConn1 -- Conn1/RConn1

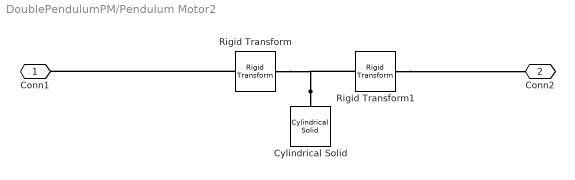
== system DoublePendulumPM/Pendulum Motor2 ==
  Cylindrical Solid : sm_lib/Body Elements/Cylindrical Solid  GraphicAmbientColor=[0.15 0.15 0.15 1.0]  BasedOnType=Density  CenterOfMass=[0 0 0]  CenterOfMassUnits=m  GraphicDiffuseColor=rgb  CylinderLength=L  CylinderLengthUnits=m  CylinderRadius=R  CylinderRadiusUnits=m  Density=rho  DensityUnits=kg/m^3  DoExposeReferenceFrame=on  GraphicEmissiveColor=[0.0 0.0 0.0 1.0]  ExportEntireGeometry=off  SerializedFrames=<Frames/>  MarkerShape=Sphere  MarkerSize=10  GraphicType=FromGeometry  InertiaType=CalculateFromGeometry  Mass=1  MassUnits=kg  MomentsOfInertia=[1 1 1]  MomentsOfInertiaUnits=kg*m^2  GraphicOpacity=1.0  ProductsOfInertia=[0 0 0]  ProductsOfInertiaUnits=kg*m^2  GraphicShininess=75  GraphicSpecularColor=[0.5 0.5 0.5 1.0]  GraphicVisPropType=SimpleVisualProperties
  Rigid Transform : sm_lib/Frames and Transforms/Rigid Transform  TranslationMethod=StandardAxis  TranslationStandardOffset=L/2  TranslationStandardOffsetUnits=m  TranslationStandardAxis=-Z  TranslationCartesianOffset=[0 0 0]  TranslationCartesianOffsetUnits=m  TranslationROffset=0  TranslationROffsetUnits=m  TranslationZOffset=0  TranslationZOffsetUnits=m  TranslationThetaOffset=0  TranslationThetaOffsetUnits=deg  RotationMethod=None  RotationAngleUnits=deg  RotationStandardAxis=-X  RotationAngle=L/2  RotationArbitraryAxis=[0 0 1]  FollAlignAxisA=-X  BaseAlignAxisA=+Y  FollAlignAxisB=+Y  BaseAlignAxisB=+Z  RotationSequenceAxes=FollowerAxes  RotationSequence=XYX  RotationSequenceAngles=[0 0 0]  RotationSequenceAnglesUnits=deg  RotationMatrix=[1 0 0; 0 1 0; 0 0 1]  Quaternion=[1 0 0 0]
  Rigid Transform1 : sm_lib/Frames and Transforms/Rigid Transform  TranslationMethod=StandardAxis  TranslationStandardOffset=L/2  TranslationStandardOffsetUnits=m  TranslationStandardAxis=+Z  TranslationCartesianOffset=[0 0 0]  TranslationCartesianOffsetUnits=m  TranslationROffset=0  TranslationROffsetUnits=m  TranslationZOffset=0  TranslationZOffsetUnits=m  TranslationThetaOffset=0  TranslationThetaOffsetUnits=deg  RotationMethod=None  RotationAngleUnits=deg  RotationStandardAxis=-X  RotationAngle=L/2  RotationArbitraryAxis=[0 0 1]  FollAlignAxisA=-X  BaseAlignAxisA=+Y  FollAlignAxisB=+Y  BaseAlignAxisB=+Z  RotationSequenceAxes=FollowerAxes  RotationSequence=XYX  RotationSequenceAngles=[0 0 0]  RotationSequenceAnglesUnits=deg  RotationMatrix=[1 0 0; 0 1 0; 0 0 1]  Quaternion=[1 0 0 0]
  Conn1 : PMIOPort  Side=Left
  Conn2 : PMIOPort  Port=2  Side=Right
  connections:
  Cylindrical Solid/RConn1 -- Rigid Transform/LConn1 -- Rigid Transform1/LConn1
  Rigid Transform1/RConn1 -- Conn2/RConn1
  Rigid Transform/RConn1 -- Conn1/RConn1

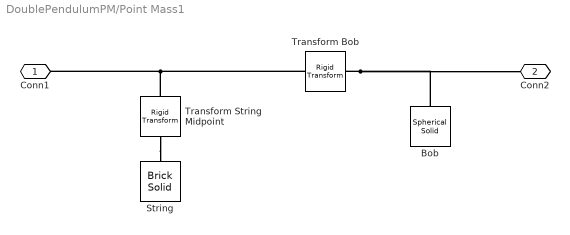
== system DoublePendulumPM/Point Mass1 ==
  Bob : sm_lib/Body Elements/Spherical Solid  GraphicAmbientColor=[0.15 0.15 0.15 1.0]  BasedOnType=Density  CenterOfMass=[0 0 0]  CenterOfMassUnits=m  GraphicDiffuseColor=rgb  Density=1000  DensityUnits=kg/(m^3)  DoExposeReferenceFrame=on  GraphicEmissiveColor=[0.0 0.0 0.0 1.0]  ExportEntireGeometry=off  SerializedExposedGeometries=<exposedGeometries/>  SerializedFrames=<Frames/>  MarkerShape=Sphere  MarkerSize=10  GraphicType=FromGeometry  InertiaType=PointMass  Mass=M  MassUnits=kg  MomentsOfInertia=[1 1 1]*1e-3  MomentsOfInertiaUnits=kg*m^2  GraphicOpacity=1.0  ProductsOfInertia=[0 0 0]  ProductsOfInertiaUnits=kg*m^2  GraphicShininess=75  GraphicSpecularColor=[0.5 0.5 0.5 1.0]  SphereRadius=0.03  SphereRadiusUnits=m  GraphicVisPropType=SimpleVisualProperties
  String : sm_lib/Body Elements/Brick Solid  GraphicAmbientColor=[0.15 0.15 0.15 1.0]  BasedOnType=Density  BrickDimensions=[ L 0.01 0.01]  BrickDimensionsUnits=m  CenterOfMass=[0 0 0]  CenterOfMassUnits=m  GraphicDiffuseColor=rgb  Density=0  DensityUnits=kg/(m^3)  DoExposeReferenceFrame=on  GraphicEmissiveColor=[0.0 0.0 0.0 1.0]  ExportEntireGeometry=off  SerializedFrames=<Frames/>  MarkerShape=Sphere  MarkerSize=10  GraphicType=FromGeometry  InertiaType=CalculateFromGeometry  Mass=0  MassUnits=kg  MomentsOfInertia=[1 1 1]*1e-3  MomentsOfInertiaUnits=kg*m^2  GraphicOpacity=1.0  ProductsOfInertia=[0 0 0]  ProductsOfInertiaUnits=kg*m^2  GraphicShininess=75  GraphicSpecularColor=[0.5 0.5 0.5 1.0]  GraphicVisPropType=SimpleVisualProperties
  "Transform Bob " : sm_lib/Frames and Transforms/Rigid Transform  TranslationMethod=StandardAxis  TranslationStandardOffset=L  TranslationStandardOffsetUnits=m  TranslationStandardAxis=+X  TranslationCartesianOffset=[0 0 0]  TranslationCartesianOffsetUnits=m  TranslationROffset=0  TranslationROffsetUnits=m  TranslationZOffset=0  TranslationZOffsetUnits=m  TranslationThetaOffset=0  TranslationThetaOffsetUnits=deg  RotationMethod=None  RotationAngleUnits=deg  RotationStandardAxis=+Z  RotationAngle=0  RotationArbitraryAxis=[0 0 1]  FollAlignAxisA=+X  BaseAlignAxisA=+Y  FollAlignAxisB=+Y  BaseAlignAxisB=+Z  RotationSequenceAxes=FollowerAxes  RotationSequence=XYX  RotationSequenceAngles=[0 0 0]  RotationSequenceAnglesUnits=deg  RotationMatrix=[1 0 0; 0 1 0; 0 0 1]  Quaternion=[1 0 0 0]
  Transform String Midpoint : sm_lib/Frames and Transforms/Rigid Transform  TranslationMethod=StandardAxis  TranslationStandardOffset=L/2  TranslationStandardOffsetUnits=m  TranslationStandardAxis=+X  TranslationCartesianOffset=[0 0 0]  TranslationCartesianOffsetUnits=m  TranslationROffset=0  TranslationROffsetUnits=m  TranslationZOffset=0  TranslationZOffsetUnits=m  TranslationThetaOffset=0  TranslationThetaOffsetUnits=deg  RotationMethod=None  RotationAngleUnits=deg  RotationStandardAxis=+Z  RotationAngle=0  RotationArbitraryAxis=[0 0 1]  FollAlignAxisA=+X  BaseAlignAxisA=+Y  FollAlignAxisB=+Y  BaseAlignAxisB=+Z  RotationSequenceAxes=FollowerAxes  RotationSequence=XYX  RotationSequenceAngles=[0 0 0]  RotationSequenceAnglesUnits=deg  RotationMatrix=[1 0 0; 0 1 0; 0 0 1]  Quaternion=[1 0 0 0]
  Conn1 : PMIOPort  Side=Left
  Conn2 : PMIOPort  Port=2  Side=Right
  connections:
  Transform String Midpoint/LConn1 -- "Transform Bob "/LConn1 -- Conn1/RConn1
  "Transform Bob "/RConn1 -- Bob/RConn1 -- Conn2/RConn1
  Transform String Midpoint/RConn1 -- String/RConn1

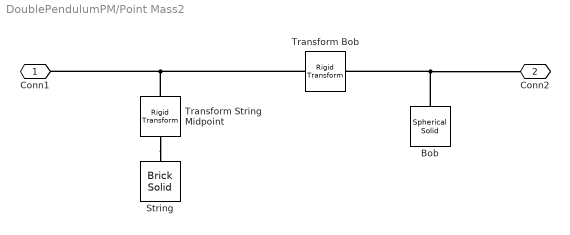
== system DoublePendulumPM/Point Mass2 ==
  Bob : sm_lib/Body Elements/Spherical Solid  GraphicAmbientColor=[0.15 0.15 0.15 1.0]  BasedOnType=Density  CenterOfMass=[0 0 0]  CenterOfMassUnits=m  GraphicDiffuseColor=rgb  Density=1000  DensityUnits=kg/(m^3)  DoExposeReferenceFrame=on  GraphicEmissiveColor=[0.0 0.0 0.0 1.0]  ExportEntireGeometry=off  SerializedExposedGeometries=<exposedGeometries/>  SerializedFrames=<Frames/>  MarkerShape=Sphere  MarkerSize=10  GraphicType=FromGeometry  InertiaType=PointMass  Mass=M  MassUnits=kg  MomentsOfInertia=[1 1 1]*1e-3  MomentsOfInertiaUnits=kg*m^2  GraphicOpacity=1.0  ProductsOfInertia=[0 0 0]  ProductsOfInertiaUnits=kg*m^2  GraphicShininess=75  GraphicSpecularColor=[0.5 0.5 0.5 1.0]  SphereRadius=0.03  SphereRadiusUnits=m  GraphicVisPropType=SimpleVisualProperties
  String : sm_lib/Body Elements/Brick Solid  GraphicAmbientColor=[0.15 0.15 0.15 1.0]  BasedOnType=Density  BrickDimensions=[ L 0.01 0.01]  BrickDimensionsUnits=m  CenterOfMass=[0 0 0]  CenterOfMassUnits=m  GraphicDiffuseColor=rgb  Density=0  DensityUnits=kg/(m^3)  DoExposeReferenceFrame=on  GraphicEmissiveColor=[0.0 0.0 0.0 1.0]  ExportEntireGeometry=off  SerializedFrames=<Frames/>  MarkerShape=Sphere  MarkerSize=10  GraphicType=FromGeometry  InertiaType=CalculateFromGeometry  Mass=0  MassUnits=kg  MomentsOfInertia=[1 1 1]*1e-3  MomentsOfInertiaUnits=kg*m^2  GraphicOpacity=1.0  ProductsOfInertia=[0 0 0]  ProductsOfInertiaUnits=kg*m^2  GraphicShininess=75  GraphicSpecularColor=[0.5 0.5 0.5 1.0]  GraphicVisPropType=SimpleVisualProperties
  "Transform Bob " : sm_lib/Frames and Transforms/Rigid Transform  TranslationMethod=StandardAxis  TranslationStandardOffset=L  TranslationStandardOffsetUnits=m  TranslationStandardAxis=+X  TranslationCartesianOffset=[0 0 0]  TranslationCartesianOffsetUnits=m  TranslationROffset=0  TranslationROffsetUnits=m  TranslationZOffset=0  TranslationZOffsetUnits=m  TranslationThetaOffset=0  TranslationThetaOffsetUnits=deg  RotationMethod=None  RotationAngleUnits=deg  RotationStandardAxis=+Z  RotationAngle=0  RotationArbitraryAxis=[0 0 1]  FollAlignAxisA=+X  BaseAlignAxisA=+Y  FollAlignAxisB=+Y  BaseAlignAxisB=+Z  RotationSequenceAxes=FollowerAxes  RotationSequence=XYX  RotationSequenceAngles=[0 0 0]  RotationSequenceAnglesUnits=deg  RotationMatrix=[1 0 0; 0 1 0; 0 0 1]  Quaternion=[1 0 0 0]
  Transform String Midpoint : sm_lib/Frames and Transforms/Rigid Transform  TranslationMethod=StandardAxis  TranslationStandardOffset=L/2  TranslationStandardOffsetUnits=m  TranslationStandardAxis=+X  TranslationCartesianOffset=[0 0 0]  TranslationCartesianOffsetUnits=m  TranslationROffset=0  TranslationROffsetUnits=m  TranslationZOffset=0  TranslationZOffsetUnits=m  TranslationThetaOffset=0  TranslationThetaOffsetUnits=deg  RotationMethod=None  RotationAngleUnits=deg  RotationStandardAxis=+Z  RotationAngle=0  RotationArbitraryAxis=[0 0 1]  FollAlignAxisA=+X  BaseAlignAxisA=+Y  FollAlignAxisB=+Y  BaseAlignAxisB=+Z  RotationSequenceAxes=FollowerAxes  RotationSequence=XYX  RotationSequenceAngles=[0 0 0]  RotationSequenceAnglesUnits=deg  RotationMatrix=[1 0 0; 0 1 0; 0 0 1]  Quaternion=[1 0 0 0]
  Conn1 : PMIOPort  Side=Left
  Conn2 : PMIOPort  Port=2  Side=Right
  connections:
  Transform String Midpoint/LConn1 -- "Transform Bob "/LConn1 -- Conn1/RConn1
  Bob/RConn1 -- "Transform Bob "/RConn1 -- Conn2/RConn1
  Transform String Midpoint/RConn1 -- String/RConn1
